simulink model "DYC_2018b"  (R2018b)
settings: Solver=VariableStepAuto  StartTime=0.0  StopTime=40  RelTol=1e-3
values from neighbouring files (symbols this model uses):
  Caf = 460    [trqvparameter.m]
  Car = 440    [trqvparameter.m]
  dwf = 1.2    [trqvparameter.m]
  dwr = 1.2    [trqvparameter.m]
  h = 0.29    [trqvparameter.m]
  i1 = 11.4    [trqvparameter.m]
  i2 = 3.4    [trqvparameter.m]
  Iz = 105    [trqvparameter.m]
  Kc = 10    [trqvparameter.m]
  Ki = 20    [trqvparameter.m]
  Kp = 30    [trqvparameter.m]
  lf = 0.761    [trqvparameter.m]
  lr = 0.831    [trqvparameter.m]
  m = 340    [trqvparameter.m]
  Rt = 0.2    [trqvparameter.m]
libraries: simulink x16, Solver_SF x1
settings Model: Creator=12045  LastModifiedBy=YJR
settings DataIOCC: ReturnWorkspaceOutputs=on
settings OptimizationCC: DefaultParameterBehavior=Inlined  EnhancedBackFolding=on  PassReuseOutputArgsAs=Individual arguments  ZeroExternalMemoryAtStartup=off  ZeroInternalMemoryAtStartup=off  OptimizeBlockOrder=speed  DifferentSizesBufferReuse=on  OptimizationCustomize=off
settings DebuggingCC: ParameterPrecisionLossMsg=none  ParameterTunabilityLossMsg=error  UnconnectedInputMsg=none  UnconnectedOutputMsg=none  UnconnectedLineMsg=none  SFMachineParentedDataDiag=error
settings ModelReferenceCC: EnableRefExpFcnMdlSchedulingChecks=off
settings SFSimCC: MATLABDynamicMemAlloc=off
settings RTWCC: SystemTargetFile=ert.tlc  TemplateMakefile=ert_default_tmf
settings CodeAppCC: ForceParamTrailComments=on  IgnoreCustomStorageClasses=off  OperatorAnnotations=on  SimulinkDataObjDesc=on  SFDataObjDesc=on  InsertBlockDesc=on
settings ERTTargetCC: TargetLangStandard=C99 (ISO)  GenerateSampleERTMain=on  InlinedParameterPlacement=NonHierarchical  ERTCustomFileTemplate=example_file_process.tlc

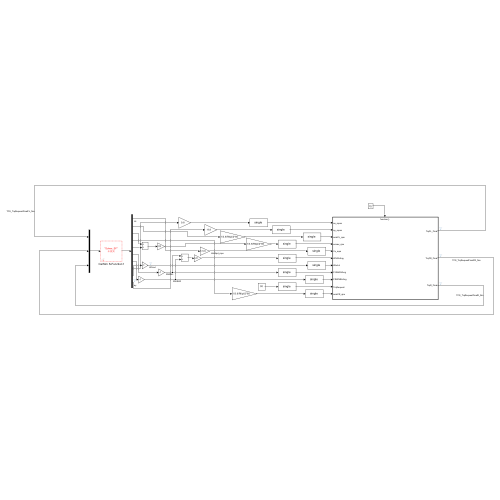
[thumbnail: Simulink's stored preview of the top-level diagram]
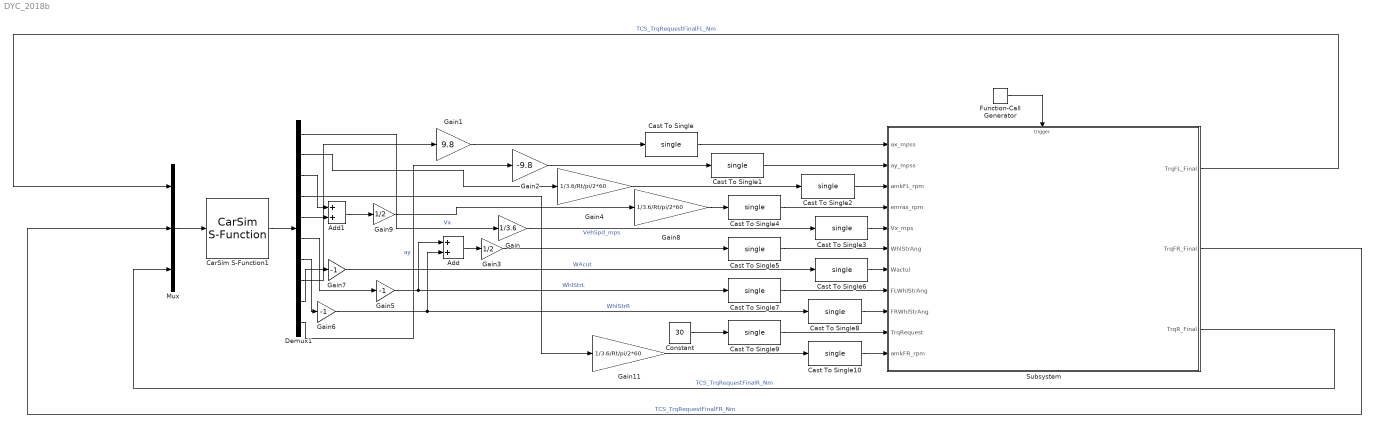
== system DYC_2018b ==
  Add : Sum
  Add1 : Sum
  CarSim S-Function1 : Solver_SF/CarSim S-Function  Priority=1  SIMFILE=simfile.sim  Run_RTs=off  vs_state_ind=Run  StopMode_ind=Vehicle Model
  Cast To Single{,1..10} (11 alike) : DataTypeConversion  OutDataTypeStr=single
  Constant : Constant  Value=30
  Demux1 : Demux  Outputs=10
  Function-Call Generator : simulink/Ports & Subsystems/Function-Call Generator  sample_time=0.01  numberOfIterations=1
  Gain : Gain  Gain=1/3.6
  Gain1 : Gain  Gain=9.8
  Gain11 : Gain  Gain=1/3.6/Rt/pi/2*60
  Gain2 : Gain  Gain=-9.8
  Gain3 : Gain  Gain=1/2
  Gain4 : Gain  Gain=1/3.6/Rt/pi/2*60
  Gain5 : Gain  Gain=-1
  Gain6 : Gain  Gain=-1
  Gain7 : Gain  Gain=-1
  Gain8 : Gain  Gain=1/3.6/Rt/pi/2*60
  Gain9 : Gain  Gain=1/2
  Mux : Mux  Inputs=3
  Subsystem : Subsystem
  wires:
  Demux1/8 -> Gain1/1
  Gain2/1 -> Cast To Single1/1
  Gain4/1 -> Cast To Single2/1
  Gain8/1 -> Cast To Single4/1
  Gain3/1 -> Cast To Single5/1
  Constant/1 -> Cast To Single9/1
  Function-Call Generator/1 -> Subsystem/Trigger
  Demux1/9 -> Gain7/1
  Demux1/10 -> Gain2/1  "ay"
  Mux/1 -> CarSim S-Function1/1
  Demux1/5 -> Add1/2
  Demux1/3 -> Add1/1
  Add1/1 -> Gain9/1
  Demux1/6 -> Gain5/1
  Subsystem/1(TrqFL_Final) -> Mux/1  "TCS_TrqRequestFinalFL_Nm"
  Demux1/7 -> Gain6/1
  Demux1/1 -> Gain/1  "Vx"
  CarSim S-Function1/1 -> Demux1/1
  Gain/1 -> Cast To Single3/1  "VehSpd_mps"
  Gain11/1 -> Cast To Single10/1
  Gain7/1 -> Cast To Single6/1  "WAcut"
  Gain1/1 -> Cast To Single/1
  Gain5/1 -> Add/1, Cast To Single7/1  "WhlStrL"
  Gain6/1 -> Add/2, Cast To Single8/1  "WhlStrR"
  Add/1 -> Gain3/1
  Demux1/4 -> Gain11/1
  Gain9/1 -> Gain8/1
  Demux1/2 -> Gain4/1
  Cast To Single/1 -> Subsystem/1(ax_mpss)
  Cast To Single1/1 -> Subsystem/2(ay_mpss)
  Cast To Single2/1 -> Subsystem/3(amkFL_rpm)
  Cast To Single3/1 -> Subsystem/5(Vx_mps)
  Cast To Single4/1 -> Subsystem/4(emrax_rpm)
  Cast To Single5/1 -> Subsystem/6(WhlStrAng)
  Cast To Single6/1 -> Subsystem/7(Wactul)
  Cast To Single7/1 -> Subsystem/8(FLWhlStrAng)
  Cast To Single8/1 -> Subsystem/9(FRWhlStrAng)
  Cast To Single9/1 -> Subsystem/10(TrqRequest)
  Cast To Single10/1 -> Subsystem/11(amkFR_rpm)
  Subsystem/2(TrqFR_Final) -> Mux/2  "TCS_TrqRequestFinalFR_Nm"
  Subsystem/3(TrqR_Final) -> Mux/3  "TCS_TrqRequestFinalR_Nm"

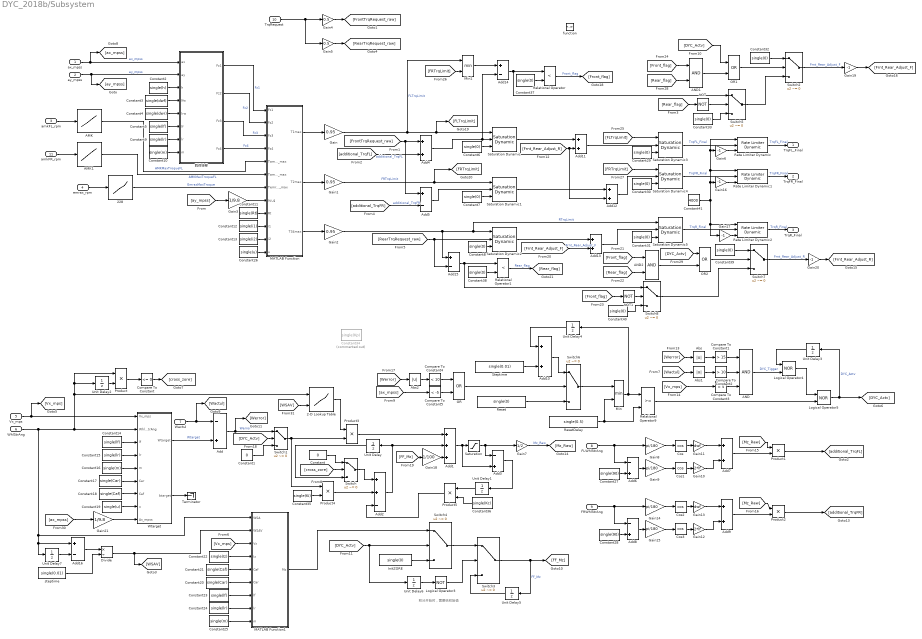
== system DYC_2018b/Subsystem ==
  note: 积分开始时，需要给初始值
  ax_mpss : Inport
  ay_mpss : Inport  Port=2
  amkFL_rpm : Inport  Port=3
  emrax_rpm : Inport  Port=4
  Vx_mps : Inport  Port=5
  WhlStrAng : Inport  Port=6
  Wactul : Inport  Port=7
  FLWhlStrAng : Inport  Port=8
  FRWhlStrAng : Inport  Port=9
  TrqRequest : Inport  Port=10
  amkFR_rpm : Inport  Port=11
  function : TriggerPort  TriggerType=function-call  VariantControl=(inherit)
  2-D Lookup Table : Lookup_n-D  BreakpointsForDimension1=[0 5 20 25]  BreakpointsForDimension2=[20 40 60]  Table=[5 7 9;5 8 12;15 9 15;15 9 15]  InternalRulePriority=Speed  RndMeth=Simplest  InputSameDT=on
  228 : Lookup_n-D  NumberOfTableDimensions=1  BreakpointsForDimension1=[200;400;600;800;1000;1200;1400;1600;1800;2000;2200;2400;2600;2800;3000;3200;3400;3600;3800;4000;4200;4400;4600;4800;5000;5200;5400]  BreakpointsForDimension2=[1:3]  Table=[229.85;229.85;229.85;229.85;229.85;229.85;229.85;229.85;229.85;229.85;229.85;229.85;229.46;229.16;228.86;228.86;228.86;228.86;228.86;227.86;227.86;226.87;225.86;224.86;220.86;218.87;215.87]  InternalRulePriority=Speed  RndMeth=Simplest  InputSameDT=on
  AMK : Lookup_n-D  NumberOfTableDimensions=1  BreakpointsForDimension1=[0;1000;2000;3000;4000;5000;6000;7000;8000;9000;10000;11000;12000;13000;14000;15000;16000;17000;18000;19000]  BreakpointsForDimension2=[1:3]  Table=[21;21;21;21;21;21;21;21;21;21;21;21;21;21;20;17.5;15;12.5;8;0]  InternalRulePriority=Speed  RndMeth=Simplest  InputSameDT=on
  AMK1 : Lookup_n-D  NumberOfTableDimensions=1  BreakpointsForDimension1=[0;1000;2000;3000;4000;5000;6000;7000;8000;9000;10000;11000;12000;13000;14000;15000;16000;17000;18000;19000]  BreakpointsForDimension2=[1:3]  Table=[21;21;21;21;21;21;21;21;21;21;21;21;21;21;20;17.5;15;12.5;8;0]  InternalRulePriority=Speed  RndMeth=Simplest  InputSameDT=on
  AND : Logic  Inputs=3  AllPortsSameDT=off  OutDataTypeStr=boolean
  AND1 : Logic  AllPortsSameDT=off  OutDataTypeStr=boolean
  AND2 : Logic  AllPortsSameDT=off  OutDataTypeStr=boolean
  Abs : Abs
  Abs1 : Abs
  Abs2 : Abs
  Add{,3,6,8} (4 alike) : Sum  Inputs=-+
  Add1 : Sum  Inputs=+++
  Add{4,7,9..13} (7 alike) : Sum
  Add{5,14..16} (4 alike) : Sum  Inputs=+-
  Add2 : Sum  Inputs=++-
  Compare To Constant : simulink/Logic and Bit Operations/Compare To Constant  relop=<=  const=0  OutDataTypeStr=boolean
  Compare To Constant1 : simulink/Logic and Bit Operations/Compare To Constant  relop=>  const=15  OutDataTypeStr=boolean
  Compare To Constant2 : simulink/Logic and Bit Operations/Compare To Constant  relop=>  const=10  OutDataTypeStr=boolean
  Compare To Constant3 : simulink/Logic and Bit Operations/Compare To Constant  relop=>  const=5  OutDataTypeStr=boolean
  Compare To Constant4 : simulink/Logic and Bit Operations/Compare To Constant  relop=<  const=10  OutDataTypeStr=boolean
  Compare To Constant5 : simulink/Logic and Bit Operations/Compare To Constant  relop=<  const=-5  OutDataTypeStr=boolean
  Constant : Constant  Value=0
  Constant1 : Constant  Value=0
  Constant10 : Constant  Value=single(m)
  Constant11 : Constant  Value=single(Rt)
  Constant12 : Constant  Value=single(i1)
  Constant13 : Constant  Value=single(i2)
  Constant14 : Constant  Value=single(lf)
  Constant15 : Constant  Value=single(lr)
  Constant16 : Constant  Value=single(m)
  Constant17 : Constant  Value=single(Car)
  Constant18 : Constant  Value=single(Caf)
  Constant19 : Constant  Value=single(u)
  Constant2 : Constant  Value=single(h)
  Constant20 : Constant  Value=single(Car)
  Constant21 : Constant  Value=single(Caf)
  Constant22 : Constant  Value=single(Iz)
  Constant23 : Constant  Value=single(lf)
  Constant24 : Constant  Value=single(lr)
  Constant25 : Constant  Value=single(m)
  Constant26 : Constant  Value=single(u)
  Constant27 : Constant  Value=single(90)
  Constant28 : Constant  Value=single(90)
  Constant{6..8,29..33,37..40} (12 alike) : Constant  Value=single(0)
  Constant3 : Constant  Value=single(dwf)
  Constant34 : Constant  Commented=on  Value=single(Kp)
  Constant35 : Constant  Value=single(Ki)
  Constant36 : Constant  Value=single(Kc)
  Constant4 : Constant  Value=single(dwr)
  Constant41 : Constant  Value=4000
  Constant5 : Constant  Value=single(lf)
  Constant9 : Constant  Value=single(lr)
  Cos{,1..3} (4 alike) : Trigonometry  Operator=cos
  Divide : Product  Inputs=*/
  Gain : Gain  Gain=0.95
  Gain1 : Gain  Gain=0.95
  Gain10 : Gain  Gain=2*lf
  Gain11 : Gain  Gain=dwf
  Gain12 : Gain  Gain=2*lf
  Gain13 : Gain  Gain=dwf
  Gain{8..9,14..15} (4 alike) : Gain  Gain=pi/180
  Gain{6,16..17,19..20} (5 alike) : Gain  Gain=-1
  Gain18 : Gain  Gain=1/100
  Gain2 : Gain  Gain=0.95
  Gain21 : Gain  Gain=1/9.8
  Gain3 : Gain  Gain=1/9.8
  Gain4 : Gain  Gain=0.5
  Gain5 : Gain  Gain=0.5
  Gain7 : Gain  Gain=1/2
  InitZORE : Constant  Value=single(0)
  Logical Operator3 : Logic  Operator=NOT  AllPortsSameDT=off  OutDataTypeStr=boolean
  Logical Operator4 : Logic  Operator=NOR  AllPortsSameDT=off  OutDataTypeStr=boolean
  Logical Operator5 : Logic  Operator=NOR  AllPortsSameDT=off  OutDataTypeStr=boolean
  MATLAB Function : MATLAB Function  TreatAsAtomicUnit=on
  MATLAB Function1 : MATLAB Function  TreatAsAtomicUnit=on
  Min : MinMax  Inputs=2
  Min1 : MinMax  Inputs=2
  NOT : Logic  Operator=NOT  AllPortsSameDT=off  OutDataTypeStr=boolean
  NOT1 : Logic  Operator=NOT  AllPortsSameDT=off  OutDataTypeStr=boolean
  OR : Logic  Operator=OR  AllPortsSameDT=off  OutDataTypeStr=boolean
  OR1 : Logic  Operator=OR  AllPortsSameDT=off  OutDataTypeStr=boolean
  OR2 : Logic  Operator=OR  AllPortsSameDT=off  OutDataTypeStr=boolean
  Product{,1..5} (6 alike) : Product
  Rate Limiter Dynamic : simulink/Discontinuities/Rate Limiter Dynamic
  Rate Limiter Dynamic1 : simulink/Discontinuities/Rate Limiter Dynamic
  Rate Limiter Dynamic2 : simulink/Discontinuities/Rate Limiter Dynamic
  Relational Operator : RelationalOperator  Operator=<  OutDataTypeStr=boolean  RndMeth=Simplest
  Relational Operator1 : RelationalOperator  Operator=<  OutDataTypeStr=boolean  RndMeth=Simplest
  Relational Operator9 : RelationalOperator  OutDataTypeStr=boolean  RndMeth=Simplest
  Reset : Constant  Value=single(0)
  ResetDelay : Constant  Value=single(0.5)
  Saturation : Saturate  UpperLimit=500  LowerLimit=-500
  Saturation Dynamic{,1..5} (6 alike) : simulink/Discontinuities/Saturation Dynamic  OutMin=[]  OutMax=[]  OutDataTypeStr=Inherit: Same as second input  OutDataType=fixdt(1, 16)  OutScaling=2^-10  DoSatur=off
  Steptime : Constant  Value=single(0.01)
  Switch{,1..8} (9 alike) : Switch  Criteria=u2 ~= 0
  Terminator : Terminator
  Unit Delay{,1..7} (8 alike) : UnitDelay  SampleTime=-1  HasFrameUpgradeWarning=on
  Wtarget : MATLAB Function  TreatAsAtomicUnit=on
  steptime : Constant  Value=single(0.01)
  载荷转移 : MATLAB Function  TreatAsAtomicUnit=on
  TrqFL_Final : Outport
  TrqFR_Final : Outport  Port=2
  TrqR_Final : Outport  Port=3
  wires:
  Product/1 -> Compare To Constant/1
  [Frnt_Rear_Adjust_F] -> Add13/2  "Frnt_Rear_Adjust_F"
  Min1/1 -> Add14/1
  Gain15/1 -> Cos3/1
  [Werror] -> Abs2/1
  Relational Operator9/1 -> Logical Operator5/2
  Add3/1 -> Unit Delay1/1
  Gain14/1 -> Cos2/1
  Constant14/1 -> Wtarget/3(lf)
  InitZORE/1 -> Switch4/3
  AND/1 -> Logical Operator4/2  "DYC_Tigger"
  Steptime/1 -> Add10/2
  Logical Operator3/1 -> Switch3/2
  MATLAB Function/1(T1max) -> Gain/1
  Saturation Dynamic1/1 -> Add12/1
  Gain12/1 -> Add9/2
  Switch2/1 -> Gain19/1  "Frnt_Rear_Adjust_F"
  Add8/1 -> Gain15/1
  Cos3/1 -> Gain12/1
  Unit Delay/1 -> Switch/3
  Add12/1 -> Saturation Dynamic4/2
  Logical Operator5/1 -> [DYC_Actv], Unit Delay3/1  "DYC_Actv"
  OR2/1 -> Switch7/2
  Cos/1 -> Gain11/1
  Unit Delay6/1 -> Logical Operator3/1
  Add4/1 -> Add14/2, Saturation Dynamic/2
  [Wactul] -> Abs1/1
  Constant5/1 -> 载荷转移/6(lf)
  Add10/1 -> Switch6/1
  Rate Limiter Dynamic2/1 -> TrqR_Final/1  "TrqR_Final"
  Saturation/1 -> Add3/1, Gain7/1
  Constant39/1 -> Switch7/1
  Add7/1 -> Product1/2
  Switch6/1 -> Min/1
  Cos2/1 -> Gain13/1
  [Vx_mps] -> Compare To Constant3/1
  Constant24/1 -> MATLAB Function1/8(lr)
  Add9/1 -> Product2/2
  Min/1 -> Unit Delay4/1, Relational Operator9/1
  Gain1/1 -> [FRTrqLimit], Saturation Dynamic1/1  "FRTrqLimit"
  [Werror] -> Abs/1
  Abs/1 -> Compare To Constant1/1
  Add/1 -> [Werror], Switch1/1  "Werror"
  Constant30/1 -> Saturation Dynamic4/3
  Constant28/1 -> Add8/2
  Unit Delay3/1 -> Logical Operator4/1
  [additional_TrqFR] -> Add5/2  "additional_TrqFR"
  Switch7/1 -> Gain20/1  "Frnt_Rear_Adjust_R"
  2-D Lookup Table/1 -> Product3/1
  Wtarget/1(Wtarget) -> Add/2  "Wtarget"
  Compare To Constant5/1 -> OR/2
  Product1/1 -> [additional_TrqFL]
  OR1/1 -> Switch2/2
  Switch1/1 -> Product4/1, Product3/2
  [DYC_Actv] -> Unit Delay6/1, Switch4/2
  Add5/1 -> Saturation Dynamic1/2
  Gain2/1 -> Add15/1, Saturation Dynamic5/1, Saturation Dynamic2/1  "RTrqLimit"
  Gain13/1 -> Add9/1
  Gain8/1 -> Cos/1
  Compare To Constant2/1 -> AND/2
  OR/1 -> Switch6/2
  Constant6/1 -> Saturation Dynamic/3
  Cos1/1 -> Gain10/1
  Abs1/1 -> Compare To Constant2/1
  Constant1/1 -> Switch1/3
  Gain4/1 -> [FrontTrqRequest_raw]
  Add2/1 -> Add1/2, Unit Delay/1
  Product2/1 -> [additional_TrqFR]
  Switch/1 -> Add2/1
  WhlStrAng/1 -> Product/1, Unit Delay2/1, 2-D Lookup Table/1, Wtarget/2(WhlStrAng), MATLAB Function1/1(WSA), Add16/1, Unit Delay7/1
  MATLAB Function/2(T2max) -> Gain1/1
  amkFL_rpm/1 -> AMK/1
  Constant35/1 -> Product4/2
  Add15/1 -> Switch8/1, Relational Operator1/1
  [ax_mpss] -> Compare To Constant5/1
  Switch3/1 -> [FF_Mz], Unit Delay5/1  "FF_Mz"
  ResetDelay/1 -> Relational Operator9/2, Min/2
  TrqRequest/1 -> Gain5/1, Gain4/1
  Abs2/1 -> Compare To Constant4/1
  Saturation Dynamic2/1 -> Add13/1
  Unit Delay5/1 -> Switch3/3
  [Rear_flag] -> NOT/1
  Compare To Constant1/1 -> AND/1
  Unit Delay4/1 -> Add10/1
  Compare To Constant4/1 -> OR/1
  Logical Operator4/1 -> Logical Operator5/1
  Constant31/1 -> Saturation Dynamic5/3
  Gain/1 -> Min1/1, [FLTrqLimit], Saturation Dynamic/1  "FLTrqLimit"
  Constant17/1 -> Wtarget/6(Car)
  Constant36/1 -> Product5/2
  Add6/1 -> Gain9/1
  Vx_mps/1 -> Wtarget/1(Vx_mps), [Vx_mps]
  Relational Operator1/1 -> [Rear_flag]  "Rear_flag"
  Unit Delay1/1 -> Product5/1
  Constant7/1 -> Saturation Dynamic1/3
  Constant29/1 -> Saturation Dynamic3/3
  Product5/1 -> Add2/3
  Add13/1 -> Saturation Dynamic5/2
  [DYC_Actv] -> OR1/1
  AND1/1 -> OR1/2
  Constant2/1 -> 载荷转移/3(h)
  [Frnt_Rear_Adjust_R] -> Add12/2, Add11/2
  Saturation Dynamic4/1 -> Rate Limiter Dynamic1/2  "TrqFR_Final"
  Compare To Constant3/1 -> AND/3
  Gain9/1 -> Cos1/1
  Add14/1 -> Relational Operator/1, Switch5/1
  FLWhlStrAng/1 -> Add6/1, Gain8/1
  Compare To Constant/1 -> [cross_zore]
  MATLAB Function1/1(Mz) -> Switch4/1
  [Mz_Raw] -> Product1/1
  emrax_rpm/1 -> 228/1
  Saturation Dynamic3/1 -> Rate Limiter Dynamic/2  "TrqFL_Final"
  Saturation Dynamic/1 -> Add11/1
  [FLTrqLimit] -> Saturation Dynamic3/1
  228/1 -> MATLAB Function/7(Temrax_max)  "EmraxMaxTroque"
  Relational Operator/1 -> [Front_flag]  "Front_flag"
  Reset/1 -> Switch6/3
  [ay_mpss] -> Gain3/1
  [FRTrqLimit] -> Min1/2
  Add11/1 -> Saturation Dynamic3/2
  Constant38/1 -> Relational Operator1/2
  [Front_flag] -> NOT1/1
  Switch5/1 -> Switch2/3
  载荷转移/4(Fz4) -> MATLAB Function/4(Fz4)  "Fz4"
  Constant37/1 -> Relational Operator/2
  Wtarget/2(btarget) -> Terminator/1
  Constant32/1 -> Switch2/1
  [FRTrqLimit] -> Saturation Dynamic4/1
  Constant18/1 -> Wtarget/7(Caf)
  [Front_flag] -> AND2/1
  Switch4/1 -> Switch3/1
  [FF_Mz] -> Gain18/1
  [Rear_flag] -> AND1/2
  [Rear_flag] -> AND2/2
  ay_mpss/1 -> 载荷转移/2(ay), [ay_mpss]  "ay_mpss"
  AND2/1 -> OR2/2
  FRWhlStrAng/1 -> Gain14/1, Add8/1
  Switch8/1 -> Switch7/3
  Add1/1 -> Saturation/1, Add3/2
  Gain5/1 -> [RearTrqRequest_raw]
  [Mz_Raw] -> Product2/1
  Constant33/1 -> Switch5/3
  [Front_flag] -> AND1/1
  Constant40/1 -> Switch8/3
  [cross_zore] -> Switch/2
  [DYC_Actv] -> OR2/1
  Gain10/1 -> Add7/2
  载荷转移/2(Fz2) -> MATLAB Function/2(Fz2)  "Fz2"
  AMK/1 -> MATLAB Function/5(TamkFL_max)  "AMKMaxTroqueFL"
  Gain11/1 -> Add7/1
  Constant3/1 -> 载荷转移/4(lfw)
  [DYC_Actv] -> Switch1/2
  Constant8/1 -> Saturation Dynamic2/3
  Constant23/1 -> MATLAB Function1/7(lf)
  Constant4/1 -> 载荷转移/5(lrw)
  Gain7/1 -> [Mz_Raw]  "Mz_Raw"
  Constant19/1 -> Wtarget/8(u)
  Constant27/1 -> Add6/2
  Constant25/1 -> MATLAB Function1/9(m)
  Wactul/1 -> Add/1, [Wactul]
  Unit Delay2/1 -> Product/2
  [FrontTrqRequest_raw] -> Add5/1, Add4/1
  Constant26/1 -> MATLAB Function/12(u)
  Constant20/1 -> MATLAB Function1/6(Car)
  Constant22/1 -> MATLAB Function1/4(Iz)
  Constant12/1 -> MATLAB Function/10(i1)
  Constant16/1 -> Wtarget/5(m)
  Constant21/1 -> MATLAB Function1/5(Caf)
  ax_mpss/1 -> [ax_mpss], 载荷转移/1(ax)  "ax_mpss"
  Constant10/1 -> 载荷转移/8(m)
  载荷转移/3(Fz3) -> MATLAB Function/3(Fz3)  "Fz3"
  载荷转移/1(Fz1) -> MATLAB Function/1(Fz1)  "Fz1"
  [Vx_mps] -> MATLAB Function1/3(Vx)
  MATLAB Function/3(T34max) -> Gain2/1
  Gain3/1 -> MATLAB Function/8(ay_g)
  Constant/1 -> Switch/1
  [RearTrqRequest_raw] -> Saturation Dynamic2/2, Add15/2
  [additional_TrqFL] -> Add4/2  "additional_TrqFL"
  Product3/1 -> Add1/1
  Product4/1 -> Add2/2
  Constant15/1 -> Wtarget/4(lr)
  Constant13/1 -> MATLAB Function/11(i2)
  Constant9/1 -> 载荷转移/7(lr)
  Constant11/1 -> MATLAB Function/9(Rt)
  Unit Delay7/1 -> Add16/2
  Add16/1 -> Divide/1
  steptime/1 -> Divide/2
  Divide/1 -> [WSAV], MATLAB Function1/2(WSAV)
  amkFR_rpm/1 -> AMK1/1
  AMK1/1 -> MATLAB Function/6(TamkFR_max)  "AMKMaxTroqueFL"
  Rate Limiter Dynamic/1 -> TrqFL_Final/1  "TrqFL_Final"
  Rate Limiter Dynamic1/1 -> TrqFR_Final/1  "TrqFR_Final"
  Saturation Dynamic5/1 -> Rate Limiter Dynamic2/2  "TrqR_Final"
  Constant41/1 -> Rate Limiter Dynamic/1, Gain6/1, Rate Limiter Dynamic1/1, Gain16/1, Gain17/1, Rate Limiter Dynamic2/1
  Gain6/1 -> Rate Limiter Dynamic/3
  Gain16/1 -> Rate Limiter Dynamic1/3
  Gain17/1 -> Rate Limiter Dynamic2/3
  Gain18/1 -> Add1/3
  NOT/1 -> Switch5/2
  NOT1/1 -> Switch8/2
  Gain19/1 -> [Frnt_Rear_Adjust_F]
  Gain20/1 -> [Frnt_Rear_Adjust_R]
  [ax_mpss] -> Gain21/1
  Gain21/1 -> Wtarget/9(Ax_mpss)
  [WSAV] -> 2-D Lookup Table/2

== matlab function DYC_2018b/Subsystem/Wtarget ==
  data: Vx_mps input size=1; Wtarget output size=1; WhlStrAng input size=1; btarget output; lf input; lr input; m input; Car input; Caf input; u input; Ax_mpss input
function [Wtarget,btarget] = fcn(Vx_mps,WhlStrAng,lf,lr,m,Car,Caf,u,Ax_mpss)
Wdes = Vx_mps*WhlStrAng/(lf+lr+(m*Vx_mps*Vx_mps*(lr*Car-lf*Caf)/Caf/Car/(lr+lf)/2));
Wu = 0.85*u*9.8/Ax_mpss;
temp = min(abs(Wu),abs(Wdes));
    Wtarget = temp*sign(Wdes);
%     Wtarget = Wdes;

bdes = (lr-lf*m*Vx_mps*Vx_mps/Car/(lf+lr)/2)*WhlStrAng/(lr+lf+m*Vx_mps*Vx_mps*(lr*Car-lf*Caf)/Car/Caf/(lf+lr)/2);
bu = atan(0.02*u*9.8);
if abs(bdes)<=bu
btarget = bdes;
else
    btarget = bu*sign(bdes);
end

== matlab function DYC_2018b/Subsystem/MATLAB Function ==
  data: Fz1 input; T1max output; Fz2 input; Fz3 input; Fz4 input; T2max output; T34max output; TamkFL_max input; TamkFR_max input; Temrax_max input; ay_g input; Rt input; i1 input; i2 input; u input
function [T1max,T2max,T34max] = fcn(Fz1,Fz2,Fz3,Fz4, TamkFL_max,TamkFR_max, Temrax_max,ay_g,Rt,i1,i2,u)
g = 9.8;

Fx1 = sqrt(power(Fz1*u,2)-power(Fz1*ay_g/g,2));
Fx2 = sqrt(power(Fz2*u,2)-power(Fz2*ay_g/g,2));
Fx3 = sqrt(power(Fz3*u,2)-power(Fz3*ay_g/g,2));
Fx4 = sqrt(power(Fz4*u,2)-power(Fz4*ay_g/g,2));


T1max = min(Fx2*Rt/i1,TamkFR_max);
T2max = min(Fx1*Rt/i1,TamkFL_max);
T34max = min((Fx4+Fx3)/2*Rt/i2,Temrax_max);

== matlab function DYC_2018b/Subsystem/MATLAB Function1 ==
  data: WSA input; Mz output; WSAV input; Vx input; Iz input; Caf input; Car input; lf input; lr input; m input
function Mz = fcn(WSA,WSAV,Vx,Iz,Caf,Car,lf,lr,m)

Mz = ((((lf*lf*Caf+lr*lr*Car)/Iz/Vx)*(-Caf/m/Vx)-((lf*Caf-lr*Car)/m/Vx/Vx-1)*(-lf*Caf/Iz))*Iz*WSA-(-Caf/m/Vx)*Iz*WSAV)/((lf*Caf-lr*Car)/m/Vx/Vx-1)/100;

== matlab function DYC_2018b/Subsystem/载荷转移 ==
  data: ax input; Fz1 output; Fz2 output; Fz3 output; Fz4 output; ay input; h input; lfw input; lrw input; lf input; lr input; m input
function [Fz1,Fz2,Fz3,Fz4] = fcn(ax,ay,h,lfw,lrw,lf,lr,m)
g = 9.8;

Fz1 = (lr/(lf+lr))*(0.5*m*g-m*ay*h/lfw)-0.5*m*ax*h/(lf+lr);
Fz2 = (lr/(lf+lr))*(0.5*m*g+m*ay*h/lfw)-0.5*m*ax*h/(lf+lr);
Fz3 = (lr/(lf+lr))*(0.5*m*g-m*ay*h/lrw)+0.5*m*ax*h/(lf+lr);
Fz4 = (lr/(lf+lr))*(0.5*m*g+m*ay*h/lrw)+0.5*m*ax*h/(lf+lr);
